simulink model "EVM"  (R2017a)
settings: Solver=VariableStepDiscrete  StartTime=0.0  StopTime=10  RelTol=1e-3
PostLoadFcn:
  | qamRefConst = [-3.00000000000000 + 3.00000000000000i
  | -3.00000000000000 + 1.00000000000000i
  | -3.00000000000000 - 1.00000000000000i
  | -3.00000000000000 - 3.00000000000000i
  | -1.00000000000000 + 3.00000000000000i
  | -1.00000000000000 + 1.00000000000000i
  | -1.00000000000000 - 1.00000000000000i
  | -1.00000000000000 - 3.00000000000000i
  | 1.00000000000000 + 3.00000000000000i
  | 1.00000000000000 + 1.00000000000000i
  | 1.00000000000000 - 1.00000000000000i
  | 1.00000000000000 - 3.00000000000000i
  | 3.00000000000000 + 3.00000000000000i
  | 3.00000000000000 + 1.00000000000000i
  | 3.00000000000000 - 1.00000000000000i
  | 3.00000000000000 - 3.00000000000000i];
undefined symbols (not defined in the file or in its folder): comm, constellation
libraries: commutil2 x2, commrflib2 x1, commrandsrc3 x1, commdigbbndam3 x1
settings Model: Creator=The MathWorks, Inc.  LastModifiedBy=Administrator
settings DataIOCC: LimitDataPoints=on  SaveFormat=Array  SaveOutput=off  SaveTime=off
settings OptimizationCC: BooleanDataType=off  DefaultParameterBehavior=Inlined  LocalBlockOutputs=off  LifeSpan=inf
settings DebuggingCC: AlgebraicLoopMsg=error  SolverPrmCheckMsg=warning  SingleTaskRateTransMsg=error  AllowSymbolicDim=off  SFUnexpectedBacktrackingDiag=warning  SFNoUnconditionalDefaultTransitionDiag=warning  SFExecutionAtInitializationDiag=none
settings HardwareCC: ProdBitPerPointer=32  ProdBitPerSizeT=32  ProdBitPerPtrDiffT=32  ProdLargestAtomicFloat=None  ProdIntDivRoundTo=Undefined  ProdEndianess=Unspecified  ProdWordSize=32  ProdHWDeviceType=32-bit Generic
settings ModelReferenceCC: PropagateSignalLabelsOutOfModel=off
settings GRTTargetCC: TargetLangStandard=C89/C90 (ANSI)  GeneratePreprocessorConditionals=Disable all
settings ConfigComp: CovMetricSettings=dw  CovHtmlReporting=on  CovSaveCumulativeToWorkspaceVar=on  CovSaveSingleToWorkspaceVar=on  CovExternalEMLEnable=off  CovSFcnEnable=off

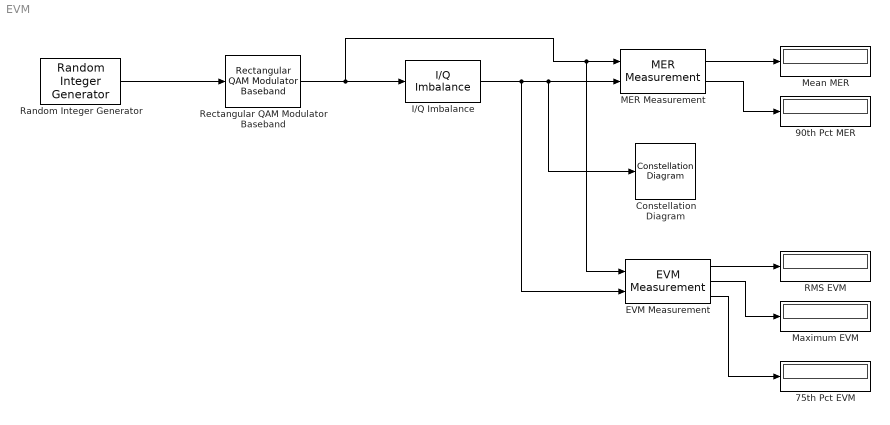
== system EVM ==
  75th Pct EVM : Display
  90th Pct MER : Display
  Constellation Diagram : ConstellationDiagram
  EVM Measurement : commutil2/EVM Measurement  Normalization=Average reference signal power  AverageConstellationPower=1  PeakConstellationPower=1  ReferenceSignalSource=Input port  ReferenceConstellation=constellation( comm.QPSKModulator )  MeasurementIntervalSource=Input length  MeasurementInterval=100  AveragingDimensions=1  MaximumEVMOutputPort=on  XPercentileEVMOutputPort=on  XPercentileValue=75  SymbolCountOutputPort=off  SimulateUsing=Interpreted execution
      settings: SourceProductName=Communications System Toolbox  SourceProductBaseCode=CM
  I/Q Imbalance : commrflib2/I//Q Imbalance  ampImbal=5  phsImbal=15  Idc=0  Qdc=0
      settings: SourceProductName=Communications System Toolbox  SourceProductBaseCode=CM
  MER Measurement : commutil2/MER Measurement  ReferenceSignalSource=Input port  ReferenceConstellation=constellation( comm.QPSKModulator )  MeasurementIntervalSource=Input length  MeasurementInterval=100  AveragingDimensions=1  MinimumMEROutputPort=off  XPercentileMEROutputPort=on  XPercentileValue=90  SymbolCountOutputPort=off  SimulateUsing=Interpreted execution
      settings: SourceProductName=Communications System Toolbox  SourceProductBaseCode=CM
  Maximum EVM : Display
  Mean MER : Display
  RMS EVM : Display
  Random Integer Generator : commrandsrc3/Random Integer Generator  SetSize=16  SeedSource=Auto  Seed=0  SampleTime=0.001  SamplesPerFrame=1000  OutputDataType=double  SimulateUsing=Interpreted execution
  Rectangular QAM Modulator Baseband : commdigbbndam3/Rectangular QAM Modulator Baseband  M=16  InType=Integer  Enc=Gray  Mapping=[0:15]  PowType=Min. distance between symbols  MinDist=2  AvgPow=1  PeakPow=1  Ph=0  outDtype=double  outWordLen=16  outUDDataType=sfix(16)  outFracLenMode=Best precision  outFracLen=15  outDataTypeStr=double  outLastDataTypeStr=double
  wires:
  Random Integer Generator/1 -> Rectangular QAM Modulator Baseband/1
  Rectangular QAM Modulator Baseband/1 -> I/Q Imbalance/1, EVM Measurement/1, MER Measurement/1
  I/Q Imbalance/1 -> EVM Measurement/2, Constellation Diagram/1, MER Measurement/2
  MER Measurement/1 -> Mean MER/1
  MER Measurement/2 -> 90th Pct MER/1
  EVM Measurement/1 -> RMS EVM/1
  EVM Measurement/2 -> Maximum EVM/1
  EVM Measurement/3 -> 75th Pct EVM/1
